simulink model "test_navigation1_1"  (R2017a)
settings: Solver=VariableStepAuto  StartTime=0.0  StopTime=inf  RelTol=1e-3
settings Model: Creator=xiaodong  LastModifiedBy=xiaodong

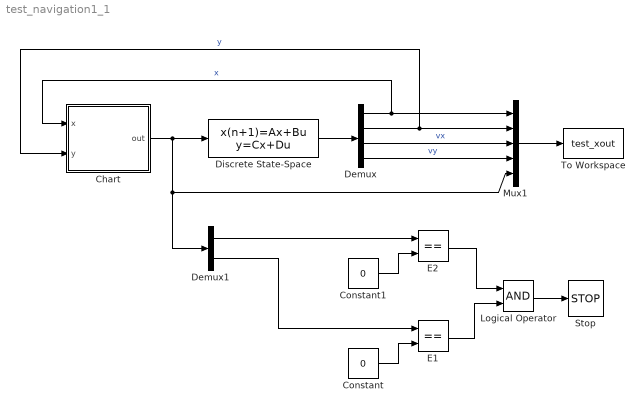
== system test_navigation1_1 ==
  Chart : Stateflow chart  TreatAsAtomicUnit=on
  Constant : Constant  Value=0
  Constant1 : Constant  Value=0
  Demux : Demux
  Demux1 : Demux  Outputs=2
  Discrete State-Space : DiscreteStateSpace  A=[1 0 0.01 0; 0 1 0 0.01; 0, 0, 0.9881, 0.0010; 0, 0, 0.0010, 0.9881]  B=[0 0; 0 0; 1 0; 0 1]  C=eye(4,4)  D=zeros(4,2)  X0="[0.300000000000000\t0.600000000000000\t0.700000000000000\t1.20000000000000]"  SampleTime=-1
  E1 : RelationalOperator  Operator===  OutDataTypeStr=boolean  RndMeth=Simplest
  E2 : RelationalOperator  Operator===  OutDataTypeStr=boolean  RndMeth=Simplest
  Logical Operator : Logic  AllPortsSameDT=off  OutDataTypeStr=boolean
  Mux1 : Mux  Inputs=5
  Stop : Stop
  To Workspace : ToWorkspace  VariableName=test_xout  SampleTime=-1
  wires:
  Chart/1(out) -> Discrete State-Space/1, Demux1/1, Mux1/5
  Discrete State-Space/1 -> Demux/1
  Demux/4 -> Mux1/4  "vy"
  Demux/3 -> Mux1/3  "vx"
  Demux/2 -> Chart/2(y), Mux1/2  "y"
  Demux/1 -> Chart/1(x), Mux1/1  "x"
  Mux1/1 -> To Workspace/1
  E2/1 -> Logical Operator/1
  E1/1 -> Logical Operator/2
  Logical Operator/1 -> Stop/1
  Constant1/1 -> E2/2
  Constant/1 -> E1/2
  Demux1/1 -> E2/1
  Demux1/2 -> E1/1

== stateflow chart test_navigation1_1/Chart ==
  state s1_1
    entry:
    out = [0.0119;  -0.0010];
    during:
    out = [0.0119;  -0.0010];
  state s2_2
    entry:
    out = [0.0010; -0.0119];
    during:
    out = [0.0010; -0.0119];
  state s3
    entry:
    out = [0.0091;   -0.0091];
    during:
    out = [0.0091;   -0.0091];
  state s2
    entry:
    out = [0.0010; -0.0119];
    during:
    out = [0.0010; -0.0119];
  state s0
    entry:
    out = [0; 0];
    during:
    out = [0; 0];
  state s1
    entry:
    out = [0.0119;  -0.0010];
    during:
    out = [0.0119;  -0.0010];
  s1_1 -> s2_2 : [-0.5011*x+0.0048*y+1<0]
  s3 -> s1_1 [order 2] : [-0.0062*x-0.4933*y+1<0]
  s2 -> s3 [order 2] : [-1.0076*x+0.0145*y+1<0]
  s3 -> s2_2 [order 3] : [-0.4973*x+0.0001*y+1<0]
  s3 -> s1 [order 1] : [-0.0034*x -1.0005*y+1>0]
  s1 -> s2 [order 1] : [ 0.0109*x-1.0004*y+1<0 ]
  s2 -> s1 [order 1] : [0.0003*x-1.0039*y+1>0]
  s2_2 -> s0 : [-0.0001*x-1.0033*y+1>0]
  (default) -> s1
  s1 -> s0 [order 2] : [-0.4985*x-0.0013*y+1<0]
  data: x input; y input; out output
